simulink model "parallel_8_prediction_and_cost_function"  (R2022a)
settings: Solver=FixedStepDiscrete  StartTime=0.0  StopTime=10.0  RelTol=1e-3
undefined symbols (not defined in the file or in its folder): f_c, L_d, L_q, L_x, L_y, p, psi_pm, R_ph
libraries: hdlsllib x10
(part 1 of 2)
settings Model: DataTypeOverride=Off  Creator=Andre Merx  LastModifiedBy=Andre Merx
settings SolverCC: AlgebraicLoopSolver=TrustRegion
settings DataIOCC: LimitDataPoints=on  SaveOutput=off  SaveTime=off
settings OptimizationCC: BlockReduction=off  ConditionallyExecuteInputs=off  DefaultParameterBehavior=Inlined  LifeSpan=inf
settings DebuggingCC: AlgebraicLoopMsg=error  SingleTaskRateTransMsg=error  UnconnectedInputMsg=warning  UnconnectedOutputMsg=warning  UnconnectedLineMsg=warning  AllowSymbolicDim=off  StrictBusMsg=ErrorOnBusTreatedAsVector  SFUnexpectedBacktrackingDiag=warning  SFNoUnconditionalDefaultTransitionDiag=warning  SFExecutionAtInitializationDiag=none  SFMachineParentedDataDiag=warning  ArithmeticOperatorsInVariantConditions=warning
settings HardwareCC: ProdBitPerPointer=32  ProdBitPerSizeT=32  ProdBitPerPtrDiffT=32  ProdLargestAtomicFloat=None  ProdIntDivRoundTo=Undefined  ProdEndianess=Unspecified  ProdWordSize=32  ProdHWDeviceType=ASIC/FPGA->ASIC/FPGA  ProdEqTarget=off
settings SFSimCC: SimUseLocalCustomCode=off  CustomCodeUndefinedFunction=UseInterfaceOnly
settings RTWCC: RTWUseLocalCustomCode=off
settings CodeAppCC: StateflowObjectComments=on
settings GRTTargetCC: TargetLangStandard=C89/C90 (ANSI)
settings ConfigComp: CovScope=ReferencedModels  CovMetricSettings=dw  CovSaveCumulativeToWorkspaceVar=on  CovSaveSingleToWorkspaceVar=on  CovExternalEMLEnable=off  CovSFcnEnable=off

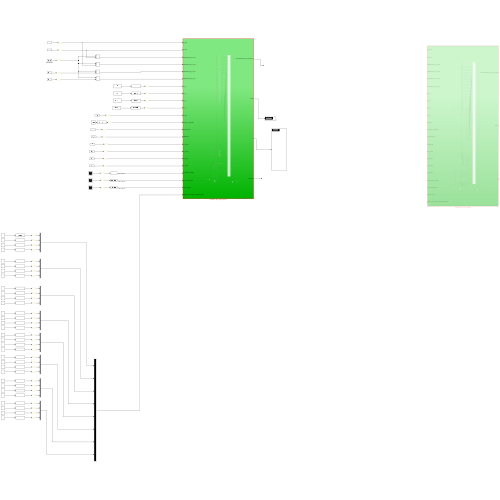
[thumbnail: Simulink's stored preview of the top-level diagram]
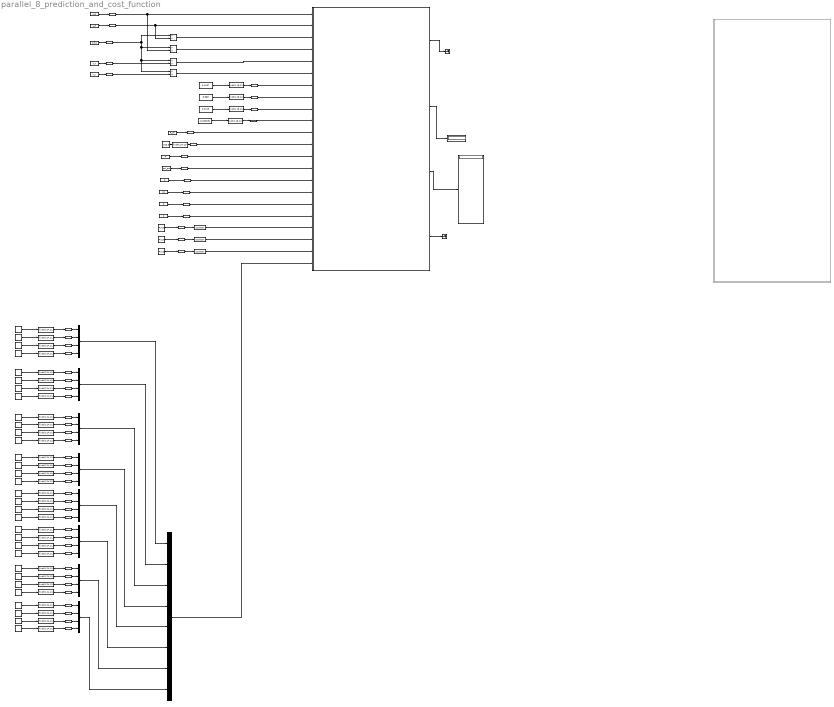
== system parallel_8_prediction_and_cost_function ==
  Constant1 : Constant  Value=L_d  OutDataTypeStr=single  SampleTime=-1
  Constant10 : Constant  Value=0  OutDataTypeStr=single  SampleTime=-1
  Constant{11,30,34,38,42,46,70,74} (8 alike) : Constant  Value=-163.1
  Constant12 : Constant  Value=L_x  OutDataTypeStr=single  SampleTime=-1
  Constant13 : Constant  Value=L_y  OutDataTypeStr=single  SampleTime=-1
  Constant18 : Constant  Value=0.4297
  Constant19 : Constant  Value=R_ph  OutDataTypeStr=single  SampleTime=-1
  Constant2 : Constant  Value=L_q  OutDataTypeStr=single  SampleTime=-1
  Constant20 : Constant  Value=313.3
  Constant21 : Constant  Value=p  OutDataTypeStr=single  SampleTime=-1
  Constant22 : Constant  Value=9.988
  Constant23 : Constant  Value=0.2219
  Constant24 : Constant  Value=psi_pm  OutDataTypeStr=single  SampleTime=-1
  Constant25 : Constant  Value=-0.003051
  Constant{4,31,35,39,43,47,71,75} (8 alike) : Constant  Value=173.9
  Constant{5,32,36,40,44,48,72,76} (8 alike) : Constant  Value=72.19
  Constant{6,33,37,41,45,49,73,77} (8 alike) : Constant  Value=-94.17
  Constant7 : Constant  Value=0  OutDataTypeStr=single  SampleTime=-1
  Constant8 : Constant  Value=10  OutDataTypeStr=single  SampleTime=-1
  Constant9 : Constant  Value=0  OutDataTypeStr=single  SampleTime=-1
  Data Type Conversion{2..6,10,20..21,25..41,62..69} (33 alike) : DataTypeConversion  OutDataTypeStr=fixdt(1,24,11)  SaturateOnIntegerOverflow=off  RndMeth=Floor
  Data Type Conversion{12..15} (4 alike) : DataTypeConversion  OutDataTypeStr=fixdt(1,18,11)  SaturateOnIntegerOverflow=off  RndMeth=Floor
  Data Type Conversion22 : DataTypeConversion  OutDataTypeStr=boolean  SaturateOnIntegerOverflow=off  RndMeth=Floor
  Data Type Conversion23 : DataTypeConversion  OutDataTypeStr=boolean  SaturateOnIntegerOverflow=off  RndMeth=Floor
  Data Type Conversion24 : DataTypeConversion  OutDataTypeStr=boolean  SaturateOnIntegerOverflow=off  RndMeth=Floor
  Display : Display
  Display1 : Display
  Divide{,1..3} (4 alike) : Product  Inputs=*/  RndMeth=Zero  SaturateOnIntegerOverflow=on
  Mux{,1..7} (8 alike) : Mux
  Mux16 : Mux  Inputs=8
  Prediction_and_cost_function1 : Subsystem  TreatAsAtomicUnit=on
  Prediction_and_cost_function2 : Subsystem  Commented=on  TreatAsAtomicUnit=on
  Pulse Generator4 : DiscretePulseGenerator  PulseType=Time based  Period=1/f_c
  Pulse Generator5 : DiscretePulseGenerator  PulseType=Time based  Period=1/f_c
  Pulse Generator6 : DiscretePulseGenerator  PulseType=Time based  Period=1/f_c
  Rate Transition{3..8,12..15,17..28,33..54,75..82} (52 alike) : RateTransition  OutPortSampleTime=Rt
  SampleTime : Constant  Value=1/f_c  OutDataTypeStr=single  SampleTime=-1
  Terminator : Terminator
  Terminator1 : Terminator
  wires:
  Mux2/1 -> Mux16/3
  Prediction_and_cost_function1/3(J) -> Display1/1
  Data Type Conversion5/1 -> Rate Transition23/1
  Data Type Conversion29/1 -> Rate Transition42/1
  Rate Transition24/1 -> Prediction_and_cost_function1/13(pole_pairs_AXI)
  Rate Transition51/1 -> Mux5/1
  Rate Transition34/1 -> Mux1/3
  Mux16/1 -> Prediction_and_cost_function1/22(dqxy_phase_voltage_per_switching_state)
  Mux6/1 -> Mux16/7
  Rate Transition22/1 -> Prediction_and_cost_function1/11(Rs_AXI)
  Constant72/1 -> Data Type Conversion63/1
  Mux1/1 -> Mux16/2
  Divide2/1 -> Prediction_and_cost_function1/5(SampleTime_div_Lx_AXI)
  Data Type Conversion2/1 -> Rate Transition4/1
  Rate Transition81/1 -> Mux6/3
  Rate Transition48/1 -> Mux3/2
  Rate Transition38/1 -> Mux1/4
  Mux/1 -> Mux16/1
  Data Type Conversion65/1 -> Rate Transition78/1
  Rate Transition44/1 -> Mux4/2
  Mux3/1 -> Mux16/4
  Rate Transition75/1 -> Mux7/1
  Divide1/1 -> Prediction_and_cost_function1/4(SampleTime_div_Lq_AXI)
  Data Type Conversion64/1 -> Rate Transition77/1
  Rate Transition4/1 -> Mux/2
  Rate Transition77/1 -> Mux7/3
  Rate Transition54/1 -> Mux5/4
  Rate Transition53/1 -> Mux5/3
  Rate Transition45/1 -> Mux4/3
  Data Type Conversion26/1 -> Rate Transition39/1
  Constant5/1 -> Data Type Conversion2/1
  Data Type Conversion3/1 -> Rate Transition18/1
  Rate Transition76/1 -> Mux7/2
  Constant42/1 -> Data Type Conversion37/1
  Rate Transition50/1 -> Mux3/4
  Data Type Conversion38/1 -> Rate Transition51/1
  Constant24/1 -> Rate Transition27/1
  Rate Transition52/1 -> Mux5/2
  Rate Transition6/1 -> Prediction_and_cost_function1/1(Lq_AXI), Divide1/2
  Rate Transition80/1 -> Mux6/2
  Rate Transition12/1 -> Prediction_and_cost_function1/15(id_ref_AXI)
  Rate Transition43/1 -> Mux4/1
  Rate Transition49/1 -> Mux3/3
  Data Type Conversion36/1 -> Rate Transition49/1
  Rate Transition47/1 -> Mux3/1
  Prediction_and_cost_function1/2(Index) -> Display/1
  Rate Transition42/1 -> Mux2/4
  Mux4/1 -> Mux16/5
  Prediction_and_cost_function1/1(done_Prediction_and_cost_function) -> Terminator/1
  Data Type Conversion23/1 -> Prediction_and_cost_function1/21(current_valid_in)  "curent_valid_in"
  Rate Transition5/1 -> Prediction_and_cost_function1/2(Ld_AXI), Divide/2
  Mux7/1 -> Mux16/8
  Rate Transition82/1 -> Mux6/4
  Constant46/1 -> Data Type Conversion41/1
  Rate Transition40/1 -> Mux2/2
  Rate Transition39/1 -> Mux2/1
  Constant9/1 -> Rate Transition14/1
  Data Type Conversion28/1 -> Rate Transition41/1
  Constant19/1 -> Rate Transition22/1
  Constant73/1 -> Data Type Conversion64/1
  Rate Transition15/1 -> Prediction_and_cost_function1/18(iy_ref_AXI)
  Constant12/1 -> Rate Transition20/1
  Constant23/1 -> Data Type Conversion14/1
  Constant37/1 -> Data Type Conversion28/1
  Data Type Conversion66/1 -> Rate Transition79/1
  Rate Transition23/1 -> Prediction_and_cost_function1/12(omega_m_measured)
  Data Type Conversion6/1 -> Rate Transition8/1
  Constant41/1 -> Data Type Conversion32/1
  Rate Transition7/1 -> Mux/3
  Constant38/1 -> Data Type Conversion33/1
  Rate Transition18/1 -> Mux1/1
  Data Type Conversion68/1 -> Rate Transition81/1
  Constant75/1 -> Data Type Conversion66/1
  Constant74/1 -> Data Type Conversion69/1
  Rate Transition25/1 -> Prediction_and_cost_function1/8(iq_k_1)
  Constant76/1 -> Data Type Conversion67/1
  Constant21/1 -> Rate Transition24/1
  Data Type Conversion63/1 -> Rate Transition76/1
  Rate Transition14/1 -> Prediction_and_cost_function1/17(ix_ref_AXI)
  Constant2/1 -> Rate Transition6/1
  Data Type Conversion13/1 -> Rate Transition25/1
  Data Type Conversion69/1 -> Rate Transition82/1
  Data Type Conversion67/1 -> Rate Transition80/1
  Data Type Conversion62/1 -> Rate Transition75/1
  Data Type Conversion4/1 -> Rate Transition7/1
  Constant70/1 -> Data Type Conversion65/1
  Constant71/1 -> Data Type Conversion62/1
  Constant40/1 -> Data Type Conversion31/1
  Constant30/1 -> Data Type Conversion25/1
  Constant33/1 -> Data Type Conversion21/1
  Rate Transition78/1 -> Mux7/4
  Rate Transition41/1 -> Mux2/3
  Rate Transition35/1 -> Data Type Conversion24/1
  Data Type Conversion12/1 -> Rate Transition17/1
  Constant32/1 -> Data Type Conversion20/1
  Constant43/1 -> Data Type Conversion34/1
  Constant44/1 -> Data Type Conversion35/1
  Constant45/1 -> Data Type Conversion36/1
  Constant48/1 -> Data Type Conversion39/1
  Data Type Conversion41/1 -> Rate Transition54/1
  Data Type Conversion37/1 -> Rate Transition50/1
  Data Type Conversion30/1 -> Rate Transition43/1
  Rate Transition79/1 -> Mux6/1
  Data Type Conversion27/1 -> Rate Transition40/1
  Data Type Conversion39/1 -> Rate Transition52/1
  Constant36/1 -> Data Type Conversion27/1
  Rate Transition3/1 -> Mux/1
  Constant11/1 -> Data Type Conversion6/1
  Data Type Conversion32/1 -> Rate Transition45/1
  Data Type Conversion33/1 -> Rate Transition46/1
  Constant34/1 -> Data Type Conversion29/1
  Data Type Conversion35/1 -> Rate Transition48/1
  Constant35/1 -> Data Type Conversion26/1
  Rate Transition46/1 -> Mux4/4
  Data Type Conversion20/1 -> Rate Transition33/1
  Data Type Conversion21/1 -> Rate Transition34/1
  Constant20/1 -> Data Type Conversion5/1
  Data Type Conversion31/1 -> Rate Transition44/1
  Data Type Conversion25/1 -> Rate Transition38/1
  Constant22/1 -> Data Type Conversion13/1
  Pulse Generator4/1 -> Rate Transition35/1
  Rate Transition19/1 -> Divide1/1, Divide3/1, Divide2/1, Divide/1
  Constant77/1 -> Data Type Conversion68/1
  Data Type Conversion14/1 -> Rate Transition26/1
  Rate Transition13/1 -> Prediction_and_cost_function1/16(iq_ref_AXI)
  Data Type Conversion34/1 -> Rate Transition47/1
  Pulse Generator5/1 -> Rate Transition36/1
  Rate Transition8/1 -> Mux/4
  Constant47/1 -> Data Type Conversion38/1
  Rate Transition36/1 -> Data Type Conversion22/1
  Pulse Generator6/1 -> Rate Transition37/1
  Rate Transition17/1 -> Prediction_and_cost_function1/7(id_k_1)
  Data Type Conversion22/1 -> Prediction_and_cost_function1/20(done_vsd_and_park)  "curent_valid_in"
  Rate Transition37/1 -> Data Type Conversion23/1
  Constant7/1 -> Rate Transition12/1
  Data Type Conversion15/1 -> Rate Transition28/1
  Rate Transition21/1 -> Divide3/2
  Rate Transition27/1 -> Prediction_and_cost_function1/14(psiPM_AXI)
  Constant39/1 -> Data Type Conversion30/1
  Data Type Conversion40/1 -> Rate Transition53/1
  Constant8/1 -> Rate Transition13/1
  Constant6/1 -> Data Type Conversion4/1
  Rate Transition26/1 -> Prediction_and_cost_function1/9(ix_k_1)
  Rate Transition28/1 -> Prediction_and_cost_function1/10(iy_k_1)
  Divide3/1 -> Prediction_and_cost_function1/6(SampleTime_div_Ly_AXI)
  Data Type Conversion10/1 -> Rate Transition3/1
  Rate Transition33/1 -> Mux1/2
  Constant31/1 -> Data Type Conversion3/1
  Constant25/1 -> Data Type Conversion15/1
  Constant1/1 -> Rate Transition5/1
  Constant10/1 -> Rate Transition15/1
  Divide/1 -> Prediction_and_cost_function1/3(SampleTime_div_Ld_AXI)
  Constant18/1 -> Data Type Conversion12/1
  Constant4/1 -> Data Type Conversion10/1
  Data Type Conversion24/1 -> Prediction_and_cost_function1/19(done_phase_voltages)  "curent_valid_in"
  Constant49/1 -> Data Type Conversion40/1
  Rate Transition20/1 -> Divide2/2
  SampleTime/1 -> Rate Transition19/1
  Constant13/1 -> Rate Transition21/1
  Mux5/1 -> Mux16/6
  Prediction_and_cost_function1/4(Index_AXI) -> Terminator1/1

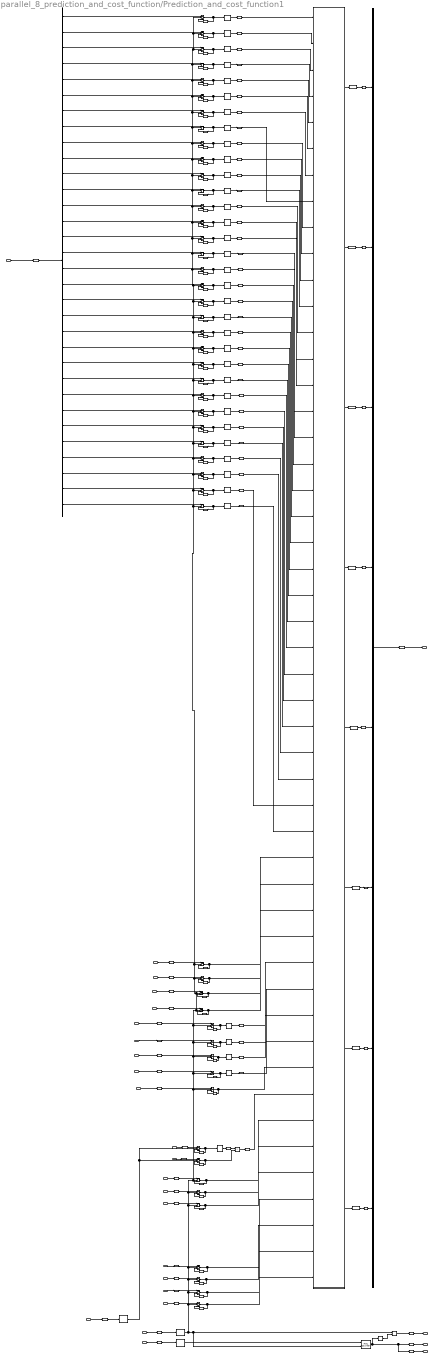
== system parallel_8_prediction_and_cost_function/Prediction_and_cost_function1 ==
  Lq_AXI : Inport
  Ld_AXI : Inport  Port=2
  SampleTime_div_Ld_AXI : Inport  Port=3
  SampleTime_div_Lq_AXI : Inport  Port=4
  SampleTime_div_Lx_AXI : Inport  Port=5
  SampleTime_div_Ly_AXI : Inport  Port=6
  id_k_1 : Inport  Port=7
  iq_k_1 : Inport  Port=8
  ix_k_1 : Inport  Port=9
  iy_k_1 : Inport  Port=10
  Rs_AXI : Inport  Port=11
  omega_m_measured : Inport  Port=12
  pole_pairs_AXI : Inport  Port=13
  psiPM_AXI : Inport  Port=14
  id_ref_AXI : Inport  Port=15
  iq_ref_AXI : Inport  Port=16
  ix_ref_AXI : Inport  Port=17
  iy_ref_AXI : Inport  Port=18
  done_phase_voltages : Inport  Port=19
  done_vsd_and_park : Inport  Port=20
  current_valid_in : Inport  Port=21
  dqxy_phase_voltage_per_switching_state : Inport  Port=22
  Compare To Constant : hdlsllib/Logic and Bit Operations/Compare To Constant  relop=<=  const=8  OutDataTypeStr=boolean
      settings: SourceProductBaseCode=SL
  Data Type Conversion{4,7..10,18,39..45,53,55..77} (37 alike) : DataTypeConversion  OutDataTypeStr=single  RndMeth=Nearest  SaturateOnIntegerOverflow=off
  Data Type Conversion{46..52,54} (8 alike) : DataTypeConversion  OutDataTypeStr=fixdt(1,20,9)  SaturateOnIntegerOverflow=off  RndMeth=Floor
  Delay{,21..32,34..37,42..45,51,57,59..60,68} (26 alike) : Delay
  Delay{1..4,8..20,33,104..135} (50 alike) : Delay  DelayLength=1
  Delay{5..7,38..41,46..50,52..56,58,61..67,69..89} (46 alike) : Delay  DelayLength=6
  Demux : Demux  Outputs=32
  Detect Rise Positive : hdlsllib/Logic and Bit Operations/Detect Rise Positive  vinit=0  OutDataTypeStr=boolean
      settings: SourceProductBaseCode=SL
  Detect Rise Positive1 : hdlsllib/Logic and Bit Operations/Detect Rise Positive  vinit=0  OutDataTypeStr=boolean
      settings: SourceProductBaseCode=SL
  Detect Rise Positive2 : hdlsllib/Logic and Bit Operations/Detect Rise Positive  vinit=0  OutDataTypeStr=boolean
      settings: SourceProductBaseCode=SL
  HDL Counter : hdlsllib/Sources/HDL Counter  CountType=Free running  CountInit=0  CountStep=1  CountMax=25  CountFromType=Initial value  CountFrom=0  CountResetPort=on  CountLoadPort=off  CountEnbPort=on  CountDirPort=off  CountHitOutputPort=off  CountDataType=Signed  CountWordLen=32  CountFracLen=0  CountSampTime=1
  Logical Operator : Logic  AllPortsSameDT=off  OutDataTypeStr=boolean
  Mux : Mux  Inputs=8
  Product : Product  Inputs=**
  Subsystem : Subsystem
  Switch_on{1..4,8..21,59..90} (50 alike) : Switch  Threshold=1  RndMeth=Simplest  SaturateOnIntegerOverflow=off  InputSameDT=off  OutDataTypeStr=Inherit: Same as first input
  done_Prediction_and_cost_function : Outport
  Index : Outport  Port=2
  J : Outport  Port=3
  Index_AXI : Outport  Port=4
  wires:
  Switch_on12/1 -> Subsystem/41(Rs15), Delay12/1
  Rs_AXI/1 -> Delay32/1
  SampleTime_div_Ld_AXI/1 -> Delay45/1
  Delay3/1 -> Switch_on3/3
  Delay10/1 -> Switch_on10/3
  iq_ref_AXI/1 -> Delay25/1
  Delay17/1 -> Switch_on18/3
  Switch_on10/1 -> Delay10/1, Subsystem/43(Lq15)
  Delay11/1 -> Switch_on11/3
  SampleTime_div_Lq_AXI/1 -> Delay44/1
  Ld_AXI/1 -> Delay28/1
  psiPM_AXI/1 -> Delay27/1
  Delay1/1 -> Switch_on1/3
  id_ref_AXI/1 -> Delay26/1
  Product/1 -> Delay6/1  "omega_el"
  Delay9/1 -> Switch_on9/3
  Delay20/1 -> Switch_on21/3
  pole_pairs_AXI/1 -> Delay30/1
  Switch_on18/1 -> Delay17/1, Subsystem/36(SampleTime_div_Ly15)
  Delay19/1 -> Switch_on20/3
  Delay13/1 -> Switch_on13/3
  Switch_on15/1 -> Delay14/1, Data Type Conversion39/1
  Delay18/1 -> Switch_on19/3
  Switch_on19/1 -> Delay18/1, Subsystem/35(SampleTime_div_Lx15)
  Switch_on20/1 -> Delay19/1, Subsystem/34(SampleTime_div_Lq15)
  Switch_on13/1 -> Delay13/1, Data Type Conversion18/1
  iy_ref_AXI/1 -> Delay23/1
  Delay2/1 -> Switch_on2/3
  Delay16/1 -> Switch_on17/3
  Switch_on17/1 -> Delay16/1, Data Type Conversion41/1
  Delay15/1 -> Switch_on16/3
  Switch_on16/1 -> Delay15/1, Data Type Conversion40/1
  Switch_on11/1 -> Data Type Conversion4/1, Delay11/1
  Delay33/1 -> Switch_on14/3
  SampleTime_div_Lx_AXI/1 -> Delay43/1
  Switch_on14/1 -> Delay33/1, Subsystem/49(iy_ref15)
  Delay12/1 -> Switch_on12/3
  done_phase_voltages/1 -> Delay21/1
  Switch_on3/1 -> Delay3/1, Subsystem/46(id_ref15)
  Switch_on21/1 -> Delay20/1, Subsystem/33(SampleTime_div_Ld15)
  Switch_on2/1 -> Delay2/1, Subsystem/47(iq_ref15)
  Lq_AXI/1 -> Delay29/1
  Switch_on1/1 -> Delay1/1, Subsystem/48(ix_ref15)
  Switch_on9/1 -> Delay9/1, Subsystem/44(Ld15)
  SampleTime_div_Ly_AXI/1 -> Delay42/1
  Delay14/1 -> Switch_on15/3
  ix_ref_AXI/1 -> Delay24/1
  Switch_on8/1 -> Delay8/1, Subsystem/45(psiPM15)
  Delay8/1 -> Switch_on8/3
  omega_m_measured/1 -> Delay31/1
  done_vsd_and_park/1 -> Delay22/1
  Detect Rise Positive1/1 -> HDL Counter/1  "End_Cycle"
  Compare To Constant/1 -> Logical Operator/2
  HDL Counter/1 -> Delay68/1, Delay60/1, Compare To Constant/1
  current_valid_in/1 -> Delay/1
  Mux/1 -> Delay57/1
  Switch_on61/1 -> Data Type Conversion9/1, Delay106/1
  Delay106/1 -> Switch_on61/3
  Delay107/1 -> Switch_on62/3
  Switch_on62/1 -> Data Type Conversion10/1, Delay107/1
  Delay104/1 -> Switch_on59/3
  Switch_on59/1 -> Data Type Conversion7/1, Delay104/1
  Delay105/1 -> Switch_on60/3
  Switch_on60/1 -> Data Type Conversion8/1, Delay105/1
  Switch_on65/1 -> Data Type Conversion44/1, Delay110/1
  Delay110/1 -> Switch_on65/3
  Delay111/1 -> Switch_on66/3
  Switch_on66/1 -> Data Type Conversion45/1, Delay111/1
  Delay108/1 -> Switch_on63/3
  Switch_on63/1 -> Data Type Conversion42/1, Delay108/1
  Delay109/1 -> Switch_on64/3
  Switch_on64/1 -> Data Type Conversion43/1, Delay109/1
  Switch_on69/1 -> Data Type Conversion56/1, Delay114/1
  Delay114/1 -> Switch_on69/3
  Delay115/1 -> Switch_on70/3
  Switch_on70/1 -> Data Type Conversion57/1, Delay115/1
  Delay112/1 -> Switch_on67/3
  Switch_on67/1 -> Data Type Conversion53/1, Delay112/1
  Delay113/1 -> Switch_on68/3
  Switch_on68/1 -> Data Type Conversion55/1, Delay113/1
  Switch_on73/1 -> Data Type Conversion60/1, Delay118/1
  Delay118/1 -> Switch_on73/3
  Delay119/1 -> Switch_on74/3
  Switch_on74/1 -> Data Type Conversion61/1, Delay119/1
  Delay116/1 -> Switch_on71/3
  Switch_on71/1 -> Data Type Conversion58/1, Delay116/1
  Delay117/1 -> Switch_on72/3
  Switch_on72/1 -> Data Type Conversion59/1, Delay117/1
  Switch_on77/1 -> Data Type Conversion64/1, Delay122/1
  Delay122/1 -> Switch_on77/3
  Delay123/1 -> Switch_on78/3
  Switch_on78/1 -> Data Type Conversion65/1, Delay123/1
  Delay120/1 -> Switch_on75/3
  Switch_on75/1 -> Data Type Conversion62/1, Delay120/1
  Delay121/1 -> Switch_on76/3
  Switch_on76/1 -> Data Type Conversion63/1, Delay121/1
  Switch_on81/1 -> Data Type Conversion68/1, Delay126/1
  Delay126/1 -> Switch_on81/3
  Delay127/1 -> Switch_on82/3
  Switch_on82/1 -> Data Type Conversion69/1, Delay127/1
  Delay124/1 -> Switch_on79/3
  Switch_on79/1 -> Data Type Conversion66/1, Delay124/1
  Delay125/1 -> Switch_on80/3
  Switch_on80/1 -> Data Type Conversion67/1, Delay125/1
  Switch_on85/1 -> Data Type Conversion72/1, Delay130/1
  Delay130/1 -> Switch_on85/3
  Delay131/1 -> Switch_on86/3
  Switch_on86/1 -> Data Type Conversion73/1, Delay131/1
  Delay128/1 -> Switch_on83/3
  Switch_on83/1 -> Data Type Conversion70/1, Delay128/1
  Delay129/1 -> Switch_on84/3
  Switch_on84/1 -> Data Type Conversion71/1, Delay129/1
  Switch_on89/1 -> Data Type Conversion76/1, Delay134/1
  Delay134/1 -> Switch_on89/3
  Delay135/1 -> Switch_on90/3
  Switch_on90/1 -> Data Type Conversion77/1, Delay135/1
  Delay132/1 -> Switch_on87/3
  Switch_on87/1 -> Data Type Conversion74/1, Delay132/1
  Delay133/1 -> Switch_on88/3
  Switch_on88/1 -> Data Type Conversion75/1, Delay133/1
  Detect Rise Positive/1 -> Logical Operator/1, HDL Counter/2, Switch_on14/2, Switch_on1/2, Switch_on8/2, Switch_on9/2, Switch_on12/2, Switch_on20/2, Switch_on90/2, Switch_on89/2, Switch_on88/2, Switch_on87/2, Switch_on86/2, Switch_on85/2, Switch_on84/2, Switch_on83/2, Switch_on82/2, Switch_on81/2, Switch_on80/2, Switch_on79/2, Switch_on78/2, Switch_on77/2, Switch_on76/2, Switch_on75/2, Switch_on74/2, Switch_on73/2, Switch_on72/2, Switch_on71/2, Switch_on70/2, Switch_on69/2, Switch_on68/2, Switch_on67/2, Switch_on66/2, Switch_on65/2, Switch_on64/2, Switch_on63/2, Switch_on62/2, Switch_on61/2, Switch_on60/2, Switch_on59/2, Switch_on21/2, Switch_on19/2, Switch_on18/2, Switch_on17/2, Switch_on16/2, Switch_on15/2, Switch_on13/2, Switch_on10/2, Switch_on3/2, Switch_on2/2  "End_Cycle"
  Logical Operator/1 -> Delay59/1
  dqxy_phase_voltage_per_switching_state/1 -> Delay51/1
  ix_k_1/1 -> Delay35/1
  iq_k_1/1 -> Delay36/1
  id_k_1/1 -> Delay37/1
  Data Type Conversion4/1 -> Delay5/1
  Demux/32 -> Switch_on59/1
  Demux/31 -> Switch_on60/1
  Demux/30 -> Switch_on61/1
  Demux/29 -> Switch_on62/1
  Demux/28 -> Switch_on63/1
  Demux/27 -> Switch_on64/1
  Demux/26 -> Switch_on65/1
  Demux/25 -> Switch_on66/1
  Demux/24 -> Switch_on67/1
  Demux/23 -> Switch_on68/1
  Demux/22 -> Switch_on69/1
  Demux/21 -> Switch_on70/1
  Demux/20 -> Switch_on71/1
  Demux/19 -> Switch_on72/1
  Demux/18 -> Switch_on73/1
  Demux/17 -> Switch_on74/1
  Demux/16 -> Switch_on75/1
  Demux/15 -> Switch_on76/1
  Demux/14 -> Switch_on77/1
  Demux/13 -> Switch_on78/1
  Demux/12 -> Switch_on79/1
  Demux/11 -> Switch_on80/1
  Demux/10 -> Switch_on81/1
  Demux/9 -> Switch_on82/1
  Demux/8 -> Switch_on83/1
  Demux/7 -> Switch_on84/1
  Demux/6 -> Switch_on85/1
  Demux/5 -> Switch_on86/1
  Demux/4 -> Switch_on87/1
  Demux/3 -> Switch_on88/1
  Demux/2 -> Switch_on89/1
  Demux/1 -> Switch_on90/1
  Detect Rise Positive2/1 -> Switch_on4/2, Switch_on11/2  "End_Cycle"
  Switch_on4/1 -> Product/2, Delay4/1
  Delay4/1 -> Switch_on4/3
  Subsystem/8(J7) -> Data Type Conversion52/1  "fc"
  Subsystem/7(J6) -> Data Type Conversion51/1  "fc"
  Subsystem/6(J5) -> Data Type Conversion50/1  "fc"
  Subsystem/5(J4) -> Data Type Conversion49/1  "fc"
  Subsystem/4(J3) -> Data Type Conversion48/1  "fc"
  Subsystem/3(J2) -> Data Type Conversion47/1  "fc"
  Subsystem/2(J1) -> Data Type Conversion46/1  "fc"
  Subsystem/1(J) -> Data Type Conversion54/1  "fc"
  Data Type Conversion54/1 -> Delay82/1  "fc"
  Data Type Conversion46/1 -> Delay83/1  "fc"
  Data Type Conversion47/1 -> Delay84/1  "fc"
  Data Type Conversion48/1 -> Delay85/1  "fc"
  Data Type Conversion49/1 -> Delay86/1  "fc"
  Data Type Conversion50/1 -> Delay87/1  "fc"
  Data Type Conversion51/1 -> Delay88/1  "fc"
  Data Type Conversion52/1 -> Delay89/1  "fc"
  Delay5/1 -> Product/1
  Delay6/1 -> Subsystem/42(omega_el15)
  iy_k_1/1 -> Delay34/1
  Data Type Conversion18/1 -> Delay7/1
  Data Type Conversion39/1 -> Delay38/1
  Data Type Conversion40/1 -> Delay39/1
  Data Type Conversion41/1 -> Delay40/1
  Delay7/1 -> Subsystem/40(iy_k_16)
  Delay38/1 -> Subsystem/39(ix_k_16)
  Delay39/1 -> Subsystem/38(iq_k_16)
  Delay40/1 -> Subsystem/37(id_k_16)
  Data Type Conversion7/1 -> Delay41/1
  Data Type Conversion8/1 -> Delay46/1
  Data Type Conversion9/1 -> Delay47/1
  Data Type Conversion10/1 -> Delay48/1
  Data Type Conversion42/1 -> Delay49/1
  Data Type Conversion43/1 -> Delay50/1
  Data Type Conversion44/1 -> Delay52/1
  Data Type Conversion45/1 -> Delay53/1
  Data Type Conversion53/1 -> Delay54/1
  Data Type Conversion55/1 -> Delay55/1
  Data Type Conversion56/1 -> Delay56/1
  Data Type Conversion57/1 -> Delay58/1
  Data Type Conversion58/1 -> Delay61/1
  Data Type Conversion59/1 -> Delay62/1
  Data Type Conversion60/1 -> Delay63/1
  Data Type Conversion61/1 -> Delay64/1
  Data Type Conversion62/1 -> Delay65/1
  Data Type Conversion63/1 -> Delay66/1
  Data Type Conversion64/1 -> Delay67/1
  Data Type Conversion65/1 -> Delay69/1
  Data Type Conversion66/1 -> Delay70/1
  Data Type Conversion67/1 -> Delay71/1
  Data Type Conversion68/1 -> Delay72/1
  Data Type Conversion69/1 -> Delay73/1
  Data Type Conversion70/1 -> Delay74/1
  Data Type Conversion71/1 -> Delay75/1
  Data Type Conversion72/1 -> Delay76/1
  Data Type Conversion73/1 -> Delay77/1
  Data Type Conversion74/1 -> Delay78/1
  Data Type Conversion75/1 -> Delay79/1
  Data Type Conversion76/1 -> Delay80/1
  Data Type Conversion77/1 -> Delay81/1
  Delay41/1 -> Subsystem/32(y_phase_voltage_per_switching_state7)
  Delay46/1 -> Subsystem/31(x_phase_voltage_per_switching_state7)
  Delay47/1 -> Subsystem/30(q_phase_voltage_per_switching_state7)
  Delay48/1 -> Subsystem/29(d_phase_voltage_per_switching_state7)
  Delay49/1 -> Subsystem/28(y_phase_voltage_per_switching_state6)
  Delay50/1 -> Subsystem/27(x_phase_voltage_per_switching_state6)
  Delay52/1 -> Subsystem/26(q_phase_voltage_per_switching_state6)
  Delay53/1 -> Subsystem/25(d_phase_voltage_per_switching_state6)
  Delay54/1 -> Subsystem/24(y_phase_voltage_per_switching_state5)
  Delay55/1 -> Subsystem/23(x_phase_voltage_per_switching_state5)
  Delay56/1 -> Subsystem/22(q_phase_voltage_per_switching_state5)
  Delay58/1 -> Subsystem/21(d_phase_voltage_per_switching_state5)
  Delay61/1 -> Subsystem/20(y_phase_voltage_per_switching_state4)
  Delay62/1 -> Subsystem/19(x_phase_voltage_per_switching_state4)
  Delay63/1 -> Subsystem/18(q_phase_voltage_per_switching_state4)
  Delay64/1 -> Subsystem/17(d_phase_voltage_per_switching_state4)
  Delay65/1 -> Subsystem/16(y_phase_voltage_per_switching_state3)
  Delay66/1 -> Subsystem/15(x_phase_voltage_per_switching_state3)
  Delay67/1 -> Subsystem/14(q_phase_voltage_per_switching_state3)
  Delay69/1 -> Subsystem/13(d_phase_voltage_per_switching_state3)
  Delay70/1 -> Subsystem/12(y_phase_voltage_per_switching_state2)
  Delay71/1 -> Subsystem/11(x_phase_voltage_per_switching_state2)
  Delay72/1 -> Subsystem/10(q_phase_voltage_per_switching_state2)
  Delay73/1 -> Subsystem/9(d_phase_voltage_per_switching_state2)
  Delay74/1 -> Subsystem/8(y_phase_voltage_per_switching_state1)
  Delay75/1 -> Subsystem/7(x_phase_voltage_per_switching_state1)
  Delay76/1 -> Subsystem/6(q_phase_voltage_per_switching_state1)
  Delay77/1 -> Subsystem/5(d_phase_voltage_per_switching_state1)
  Delay78/1 -> Subsystem/4(y_phase_voltage_per_switching_state)
  Delay79/1 -> Subsystem/3(x_phase_voltage_per_switching_state)
  Delay80/1 -> Subsystem/2(q_phase_voltage_per_switching_state)
  Delay81/1 -> Subsystem/1(d_phase_voltage_per_switching_state)
  Delay82/1 -> Mux/1
  Delay83/1 -> Mux/2
  Delay84/1 -> Mux/3
  Delay85/1 -> Mux/4
  Delay86/1 -> Mux/5
  Delay87/1 -> Mux/6
  Delay88/1 -> Mux/7
  Delay89/1 -> Mux/8
  Delay/1 -> Detect Rise Positive2/1
  Delay21/1 -> Detect Rise Positive/1
  Delay22/1 -> Detect Rise Positive1/1
  Delay23/1 -> Switch_on14/1
  Delay24/1 -> Switch_on1/1
  Delay25/1 -> Switch_on2/1
  Delay26/1 -> Switch_on3/1
  Delay27/1 -> Switch_on8/1
  Delay28/1 -> Switch_on9/1
  Delay29/1 -> Switch_on10/1
  Delay30/1 -> Switch_on4/1
  Delay31/1 -> Switch_on11/1
  Delay32/1 -> Switch_on12/1
  Delay34/1 -> Switch_on13/1
  Delay35/1 -> Switch_on15/1
  Delay36/1 -> Switch_on16/1
  Delay37/1 -> Switch_on17/1
  Delay42/1 -> Switch_on18/1
  Delay43/1 -> Switch_on19/1
  Delay44/1 -> Switch_on20/1
  Delay45/1 -> Switch_on21/1
  Delay51/1 -> Demux/1
  Delay57/1 -> J/1
  Delay59/1 -> done_Prediction_and_cost_function/1
  Delay60/1 -> Index/1
  Delay68/1 -> Index_AXI/1

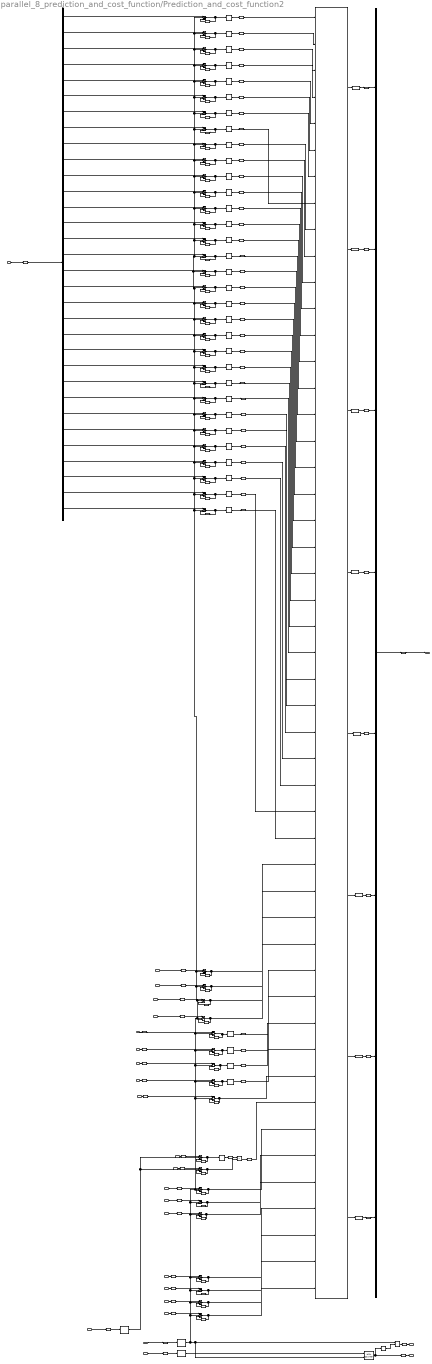
== system parallel_8_prediction_and_cost_function/Prediction_and_cost_function2 ==
  Lq_AXI : Inport
  Ld_AXI : Inport  Port=2
  SampleTime_div_Ld_AXI : Inport  Port=3
  SampleTime_div_Lq_AXI : Inport  Port=4
  SampleTime_div_Lx_AXI : Inport  Port=5
  SampleTime_div_Ly_AXI : Inport  Port=6
  id_k_1 : Inport  Port=7
  iq_k_1 : Inport  Port=8
  ix_k_1 : Inport  Port=9
  iy_k_1 : Inport  Port=10
  Rs_AXI : Inport  Port=11
  omega_m_measured : Inport  Port=12
  pole_pairs_AXI : Inport  Port=13
  psiPM_AXI : Inport  Port=14
  id_ref_AXI : Inport  Port=15
  iq_ref_AXI : Inport  Port=16
  ix_ref_AXI : Inport  Port=17
  iy_ref_AXI : Inport  Port=18
  done_phase_voltages : Inport  Port=19
  done_vsd_and_park : Inport  Port=20
  current_valid_in : Inport  Port=21
  dqxy_phase_voltage_per_switching_state : Inport  Port=22
  Compare To Constant : hdlsllib/Logic and Bit Operations/Compare To Constant  relop=<=  const=8  OutDataTypeStr=boolean
      settings: SourceProductBaseCode=SL
  Data Type Conversion{4,7..10,18,39..45,53,55..77} (37 alike) : DataTypeConversion  OutDataTypeStr=single  RndMeth=Nearest  SaturateOnIntegerOverflow=off
  Data Type Conversion{46..52,54} (8 alike) : DataTypeConversion  OutDataTypeStr=fixdt(1,20,9)  SaturateOnIntegerOverflow=off  RndMeth=Floor
  Delay{1..4,8..37,42..45,51,57,59..60,68,104..135} (75 alike) : Delay  DelayLength=1
  Delay{5..7,38..41,46..50,52..56,58,61..67,69..89} (46 alike) : Delay  DelayLength=6
  Demux : Demux  Outputs=32
  Detect Rise Positive : hdlsllib/Logic and Bit Operations/Detect Rise Positive  vinit=0  OutDataTypeStr=boolean
      settings: SourceProductBaseCode=SL
  Detect Rise Positive1 : hdlsllib/Logic and Bit Operations/Detect Rise Positive  vinit=0  OutDataTypeStr=boolean
      settings: SourceProductBaseCode=SL
  Detect Rise Positive2 : hdlsllib/Logic and Bit Operations/Detect Rise Positive  vinit=0  OutDataTypeStr=boolean
      settings: SourceProductBaseCode=SL
  HDL Counter : hdlsllib/Sources/HDL Counter  CountType=Free running  CountInit=0  CountStep=1  CountMax=25  CountFromType=Initial value  CountFrom=0  CountResetPort=on  CountLoadPort=off  CountEnbPort=on  CountDirPort=off  CountHitOutputPort=off  CountDataType=Signed  CountWordLen=32  CountFracLen=0  CountSampTime=1
  Logical Operator : Logic  AllPortsSameDT=off  OutDataTypeStr=boolean
  Mux : Mux  Inputs=8
  Product : Product  Inputs=**
  Subsystem : Subsystem
  Switch_on{1..4,8..21,59..90} (50 alike) : Switch  Threshold=1  RndMeth=Simplest  SaturateOnIntegerOverflow=off  InputSameDT=off  OutDataTypeStr=Inherit: Same as first input
  done_Prediction_and_cost_function : Outport
  Index : Outport  Port=2
  J : Outport  Port=3
  wires:
  Switch_on12/1 -> Subsystem/41(Rs15), Delay12/1
  Rs_AXI/1 -> Delay31/1
  Delay31/1 -> Switch_on12/1
  Delay23/1 -> Switch_on21/1
  Delay3/1 -> Switch_on3/3
  Delay10/1 -> Switch_on10/3
  Delay43/1 -> Switch_on2/1
  Delay17/1 -> Switch_on18/3
  Switch_on10/1 -> Delay10/1, Subsystem/43(Lq15)
  Delay11/1 -> Switch_on11/3
  Delay24/1 -> Switch_on20/1
  Delay36/1 -> Switch_on9/1
  Delay37/1 -> Switch_on8/1
  Delay1/1 -> Switch_on1/3
  Delay42/1 -> Switch_on3/1
  Product/1 -> Delay6/1  "omega_el"
  done_phase_voltages/1 -> Delay21/1
  Delay9/1 -> Switch_on9/3
  iy_k_1/1 -> Delay30/1
  Delay20/1 -> Switch_on21/3
  Delay35/1 -> Switch_on4/1
  pole_pairs_AXI/1 -> Delay35/1
  omega_m_measured/1 -> Delay51/1
  Switch_on18/1 -> Delay17/1, Subsystem/36(SampleTime_div_Ly15)
  Delay19/1 -> Switch_on20/3
  Delay13/1 -> Switch_on13/3
  Switch_on15/1 -> Delay14/1, Data Type Conversion39/1
  Delay18/1 -> Switch_on19/3
  Lq_AXI/1 -> Delay34/1
  Switch_on19/1 -> Delay18/1, Subsystem/35(SampleTime_div_Lx15)
  Switch_on20/1 -> Delay19/1, Subsystem/34(SampleTime_div_Lq15)
  Switch_on13/1 -> Delay13/1, Data Type Conversion18/1
  ix_k_1/1 -> Delay29/1
  Delay45/1 -> Switch_on14/1
  Delay2/1 -> Switch_on2/3
  Delay16/1 -> Switch_on17/3
  Switch_on17/1 -> Delay16/1, Data Type Conversion41/1
  iq_k_1/1 -> Delay28/1
  Delay15/1 -> Switch_on16/3
  Switch_on16/1 -> Delay15/1, Data Type Conversion40/1
  iq_ref_AXI/1 -> Delay43/1
  Switch_on11/1 -> Data Type Conversion4/1, Delay11/1
  Delay33/1 -> Switch_on14/3
  Ld_AXI/1 -> Delay36/1
  Delay25/1 -> Switch_on19/1
  psiPM_AXI/1 -> Delay37/1
  Switch_on14/1 -> Delay33/1, Subsystem/49(iy_ref15)
  Delay12/1 -> Switch_on12/3
  Delay21/1 -> Detect Rise Positive/1
  Switch_on3/1 -> Delay3/1, Subsystem/46(id_ref15)
  Switch_on21/1 -> Delay20/1, Subsystem/33(SampleTime_div_Ld15)
  Switch_on2/1 -> Delay2/1, Subsystem/47(iq_ref15)
  Delay34/1 -> Switch_on10/1
  iy_ref_AXI/1 -> Delay45/1
  Switch_on1/1 -> Delay1/1, Subsystem/48(ix_ref15)
  id_k_1/1 -> Delay27/1
  ix_ref_AXI/1 -> Delay44/1
  Switch_on9/1 -> Delay9/1, Subsystem/44(Ld15)
  Delay26/1 -> Switch_on18/1
  Delay14/1 -> Switch_on15/3
  id_ref_AXI/1 -> Delay42/1
  Delay44/1 -> Switch_on1/1
  Switch_on8/1 -> Delay8/1, Subsystem/45(psiPM15)
  Delay8/1 -> Switch_on8/3
  Delay51/1 -> Switch_on11/1
  SampleTime_div_Ld_AXI/1 -> Delay23/1
  SampleTime_div_Lq_AXI/1 -> Delay24/1
  SampleTime_div_Lx_AXI/1 -> Delay25/1
  SampleTime_div_Ly_AXI/1 -> Delay26/1
  done_vsd_and_park/1 -> Delay57/1
  Delay57/1 -> Detect Rise Positive1/1
  Detect Rise Positive1/1 -> HDL Counter/1  "End_Cycle"
  HDL Counter/1 -> Compare To Constant/1, Delay59/1
  Compare To Constant/1 -> Logical Operator/2
  Logical Operator/1 -> Delay22/1
  Delay59/1 -> Index/1
  current_valid_in/1 -> Delay60/1
  Delay60/1 -> Detect Rise Positive2/1
  Mux/1 -> Delay68/1
  Delay68/1 -> J/1
  Switch_on61/1 -> Data Type Conversion9/1, Delay106/1
  Delay106/1 -> Switch_on61/3
  Delay107/1 -> Switch_on62/3
  Switch_on62/1 -> Data Type Conversion10/1, Delay107/1
  Delay104/1 -> Switch_on59/3
  Switch_on59/1 -> Data Type Conversion7/1, Delay104/1
  Delay105/1 -> Switch_on60/3
  Switch_on60/1 -> Data Type Conversion8/1, Delay105/1
  Switch_on65/1 -> Data Type Conversion44/1, Delay110/1
  Delay110/1 -> Switch_on65/3
  Delay111/1 -> Switch_on66/3
  Switch_on66/1 -> Data Type Conversion45/1, Delay111/1
  Delay108/1 -> Switch_on63/3
  Switch_on63/1 -> Data Type Conversion42/1, Delay108/1
  Delay109/1 -> Switch_on64/3
  Switch_on64/1 -> Data Type Conversion43/1, Delay109/1
  Switch_on69/1 -> Data Type Conversion56/1, Delay114/1
  Delay114/1 -> Switch_on69/3
  Delay115/1 -> Switch_on70/3
  Switch_on70/1 -> Data Type Conversion57/1, Delay115/1
  Delay112/1 -> Switch_on67/3
  Switch_on67/1 -> Data Type Conversion53/1, Delay112/1
  Delay113/1 -> Switch_on68/3
  Switch_on68/1 -> Data Type Conversion55/1, Delay113/1
  Switch_on73/1 -> Data Type Conversion60/1, Delay118/1
  Delay118/1 -> Switch_on73/3
  Delay119/1 -> Switch_on74/3
  Switch_on74/1 -> Data Type Conversion61/1, Delay119/1
  Delay116/1 -> Switch_on71/3
  Switch_on71/1 -> Data Type Conversion58/1, Delay116/1
  Delay117/1 -> Switch_on72/3
  Switch_on72/1 -> Data Type Conversion59/1, Delay117/1
  Switch_on77/1 -> Data Type Conversion64/1, Delay122/1
  Delay122/1 -> Switch_on77/3
  Delay123/1 -> Switch_on78/3
  Switch_on78/1 -> Data Type Conversion65/1, Delay123/1
  Delay120/1 -> Switch_on75/3
  Switch_on75/1 -> Data Type Conversion62/1, Delay120/1
  Delay121/1 -> Switch_on76/3
  Switch_on76/1 -> Data Type Conversion63/1, Delay121/1
  Switch_on81/1 -> Data Type Conversion68/1, Delay126/1
  Delay126/1 -> Switch_on81/3
  Delay127/1 -> Switch_on82/3
  Switch_on82/1 -> Data Type Conversion69/1, Delay127/1
  Delay124/1 -> Switch_on79/3
  Switch_on79/1 -> Data Type Conversion66/1, Delay124/1
  Delay125/1 -> Switch_on80/3
  Switch_on80/1 -> Data Type Conversion67/1, Delay125/1
  Switch_on85/1 -> Data Type Conversion72/1, Delay130/1
  Delay130/1 -> Switch_on85/3
  Delay131/1 -> Switch_on86/3
  Switch_on86/1 -> Data Type Conversion73/1, Delay131/1
  Delay128/1 -> Switch_on83/3
  Switch_on83/1 -> Data Type Conversion70/1, Delay128/1
  Delay129/1 -> Switch_on84/3
  Switch_on84/1 -> Data Type Conversion71/1, Delay129/1
  Switch_on89/1 -> Data Type Conversion76/1, Delay134/1
  Delay134/1 -> Switch_on89/3
  Delay135/1 -> Switch_on90/3
  Switch_on90/1 -> Data Type Conversion77/1, Delay135/1
  Delay132/1 -> Switch_on87/3
  Switch_on87/1 -> Data Type Conversion74/1, Delay132/1
  Delay133/1 -> Switch_on88/3
  Switch_on88/1 -> Data Type Conversion75/1, Delay133/1
  Detect Rise Positive/1 -> Logical Operator/1, HDL Counter/2, Switch_on14/2, Switch_on1/2, Switch_on8/2, Switch_on9/2, Switch_on12/2, Switch_on20/2, Switch_on90/2, Switch_on89/2, Switch_on88/2, Switch_on87/2, Switch_on86/2, Switch_on85/2, Switch_on84/2, Switch_on83/2, Switch_on82/2, Switch_on81/2, Switch_on80/2, Switch_on79/2, Switch_on78/2, Switch_on77/2, Switch_on76/2, Switch_on75/2, Switch_on74/2, Switch_on73/2, Switch_on72/2, Switch_on71/2, Switch_on70/2, Switch_on69/2, Switch_on68/2, Switch_on67/2, Switch_on66/2, Switch_on65/2, Switch_on64/2, Switch_on63/2, Switch_on62/2, Switch_on61/2, Switch_on60/2, Switch_on59/2, Switch_on21/2, Switch_on19/2, Switch_on18/2, Switch_on17/2, Switch_on16/2, Switch_on15/2, Switch_on13/2, Switch_on10/2, Switch_on3/2, Switch_on2/2  "End_Cycle"
  dqxy_phase_voltage_per_switching_state/1 -> Delay32/1
  Delay22/1 -> done_Prediction_and_cost_function/1
  Delay32/1 -> Demux/1
  Delay29/1 -> Switch_on15/1
  Delay28/1 -> Switch_on16/1
  Delay27/1 -> Switch_on17/1
  Data Type Conversion4/1 -> Delay5/1
  Demux/32 -> Switch_on59/1
  Demux/31 -> Switch_on60/1
  Demux/30 -> Switch_on61/1
  Demux/29 -> Switch_on62/1
  Demux/28 -> Switch_on63/1
  Demux/27 -> Switch_on64/1
  Demux/26 -> Switch_on65/1
  Demux/25 -> Switch_on66/1
  Demux/24 -> Switch_on67/1
  Demux/23 -> Switch_on68/1
  Demux/22 -> Switch_on69/1
  Demux/21 -> Switch_on70/1
  Demux/20 -> Switch_on71/1
  Demux/19 -> Switch_on72/1
  Demux/18 -> Switch_on73/1
  Demux/17 -> Switch_on74/1
  Demux/16 -> Switch_on75/1
  Demux/15 -> Switch_on76/1
  Demux/14 -> Switch_on77/1
  Demux/13 -> Switch_on78/1
  Demux/12 -> Switch_on79/1
  Demux/11 -> Switch_on80/1
  Demux/10 -> Switch_on81/1
  Demux/9 -> Switch_on82/1
  Demux/8 -> Switch_on83/1
  Demux/7 -> Switch_on84/1
  Demux/6 -> Switch_on85/1
  Demux/5 -> Switch_on86/1
  Demux/4 -> Switch_on87/1
  Demux/3 -> Switch_on88/1
  Demux/2 -> Switch_on89/1
  Demux/1 -> Switch_on90/1
  Detect Rise Positive2/1 -> Switch_on4/2, Switch_on11/2  "End_Cycle"
  Switch_on4/1 -> Product/2, Delay4/1
  Delay4/1 -> Switch_on4/3
  Subsystem/8(J7) -> Data Type Conversion52/1  "fc"
  Subsystem/7(J6) -> Data Type Conversion51/1  "fc"
  Subsystem/6(J5) -> Data Type Conversion50/1  "fc"
  Subsystem/5(J4) -> Data Type Conversion49/1  "fc"
  Subsystem/4(J3) -> Data Type Conversion48/1  "fc"
  Subsystem/3(J2) -> Data Type Conversion47/1  "fc"
  Subsystem/2(J1) -> Data Type Conversion46/1  "fc"
  Subsystem/1(J) -> Data Type Conversion54/1  "fc"
  Data Type Conversion54/1 -> Delay82/1  "fc"
  Data Type Conversion46/1 -> Delay83/1  "fc"
  Data Type Conversion47/1 -> Delay84/1  "fc"
  Data Type Conversion48/1 -> Delay85/1  "fc"
  Data Type Conversion49/1 -> Delay86/1  "fc"
  Data Type Conversion50/1 -> Delay87/1  "fc"
  Data Type Conversion51/1 -> Delay88/1  "fc"
  Data Type Conversion52/1 -> Delay89/1  "fc"
  Delay5/1 -> Product/1
  Delay6/1 -> Subsystem/42(omega_el15)
  Delay30/1 -> Switch_on13/1
  Data Type Conversion18/1 -> Delay7/1
  Data Type Conversion39/1 -> Delay38/1
  Data Type Conversion40/1 -> Delay39/1
  Data Type Conversion41/1 -> Delay40/1
  Delay7/1 -> Subsystem/40(iy_k_16)
  Delay38/1 -> Subsystem/39(ix_k_16)
  Delay39/1 -> Subsystem/38(iq_k_16)
  Delay40/1 -> Subsystem/37(id_k_16)
  Data Type Conversion7/1 -> Delay41/1
  Data Type Conversion8/1 -> Delay46/1
  Data Type Conversion9/1 -> Delay47/1
  Data Type Conversion10/1 -> Delay48/1
  Data Type Conversion42/1 -> Delay49/1
  Data Type Conversion43/1 -> Delay50/1
  Data Type Conversion44/1 -> Delay52/1
  Data Type Conversion45/1 -> Delay53/1
  Data Type Conversion53/1 -> Delay54/1
  Data Type Conversion55/1 -> Delay55/1
  Data Type Conversion56/1 -> Delay56/1
  Data Type Conversion57/1 -> Delay58/1
  Data Type Conversion58/1 -> Delay61/1
  Data Type Conversion59/1 -> Delay62/1
  Data Type Conversion60/1 -> Delay63/1
  Data Type Conversion61/1 -> Delay64/1
  Data Type Conversion62/1 -> Delay65/1
  Data Type Conversion63/1 -> Delay66/1
  Data Type Conversion64/1 -> Delay67/1
  Data Type Conversion65/1 -> Delay69/1
  Data Type Conversion66/1 -> Delay70/1
  Data Type Conversion67/1 -> Delay71/1
  Data Type Conversion68/1 -> Delay72/1
  Data Type Conversion69/1 -> Delay73/1
  Data Type Conversion70/1 -> Delay74/1
  Data Type Conversion71/1 -> Delay75/1
  Data Type Conversion72/1 -> Delay76/1
  Data Type Conversion73/1 -> Delay77/1
  Data Type Conversion74/1 -> Delay78/1
  Data Type Conversion75/1 -> Delay79/1
  Data Type Conversion76/1 -> Delay80/1
  Data Type Conversion77/1 -> Delay81/1
  Delay41/1 -> Subsystem/32(y_phase_voltage_per_switching_state7)
  Delay46/1 -> Subsystem/31(x_phase_voltage_per_switching_state7)
  Delay47/1 -> Subsystem/30(q_phase_voltage_per_switching_state7)
  Delay48/1 -> Subsystem/29(d_phase_voltage_per_switching_state7)
  Delay49/1 -> Subsystem/28(y_phase_voltage_per_switching_state6)
  Delay50/1 -> Subsystem/27(x_phase_voltage_per_switching_state6)
  Delay52/1 -> Subsystem/26(q_phase_voltage_per_switching_state6)
  Delay53/1 -> Subsystem/25(d_phase_voltage_per_switching_state6)
  Delay54/1 -> Subsystem/24(y_phase_voltage_per_switching_state5)
  Delay55/1 -> Subsystem/23(x_phase_voltage_per_switching_state5)
  Delay56/1 -> Subsystem/22(q_phase_voltage_per_switching_state5)
  Delay58/1 -> Subsystem/21(d_phase_voltage_per_switching_state5)
  Delay61/1 -> Subsystem/20(y_phase_voltage_per_switching_state4)
  Delay62/1 -> Subsystem/19(x_phase_voltage_per_switching_state4)
  Delay63/1 -> Subsystem/18(q_phase_voltage_per_switching_state4)
  Delay64/1 -> Subsystem/17(d_phase_voltage_per_switching_state4)
  Delay65/1 -> Subsystem/16(y_phase_voltage_per_switching_state3)
  Delay66/1 -> Subsystem/15(x_phase_voltage_per_switching_state3)
  Delay67/1 -> Subsystem/14(q_phase_voltage_per_switching_state3)
  Delay69/1 -> Subsystem/13(d_phase_voltage_per_switching_state3)
  Delay70/1 -> Subsystem/12(y_phase_voltage_per_switching_state2)
  Delay71/1 -> Subsystem/11(x_phase_voltage_per_switching_state2)
  Delay72/1 -> Subsystem/10(q_phase_voltage_per_switching_state2)
  Delay73/1 -> Subsystem/9(d_phase_voltage_per_switching_state2)
  Delay74/1 -> Subsystem/8(y_phase_voltage_per_switching_state1)
  Delay75/1 -> Subsystem/7(x_phase_voltage_per_switching_state1)
  Delay76/1 -> Subsystem/6(q_phase_voltage_per_switching_state1)
  Delay77/1 -> Subsystem/5(d_phase_voltage_per_switching_state1)
  Delay78/1 -> Subsystem/4(y_phase_voltage_per_switching_state)
  Delay79/1 -> Subsystem/3(x_phase_voltage_per_switching_state)
  Delay80/1 -> Subsystem/2(q_phase_voltage_per_switching_state)
  Delay81/1 -> Subsystem/1(d_phase_voltage_per_switching_state)
  Delay82/1 -> Mux/1
  Delay83/1 -> Mux/2
  Delay84/1 -> Mux/3
  Delay85/1 -> Mux/4
  Delay86/1 -> Mux/5
  Delay87/1 -> Mux/6
  Delay88/1 -> Mux/7
  Delay89/1 -> Mux/8
